simulink subsystem "Wind_Table"  (R2023b)
settings: Solver=VariableStepAuto  StartTime=0.0  StopTime=10.0  RelTol=1e-3
undefined symbols (not defined in the file): time0, wind_direction_table, wind_speed_table
libraries: sharedtransform x1
settings Model: Creator=thatf  LastModifiedBy=thatf

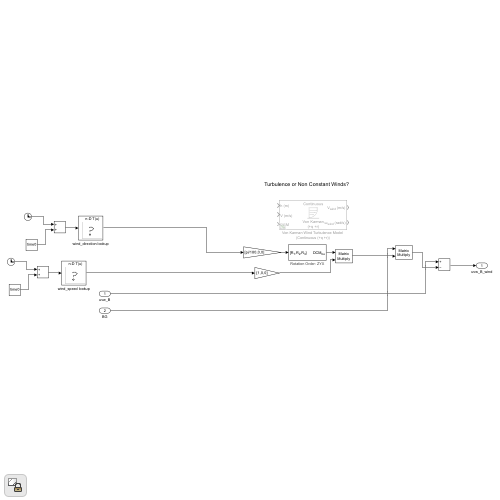
[thumbnail: Simulink's stored preview of the top-level diagram]
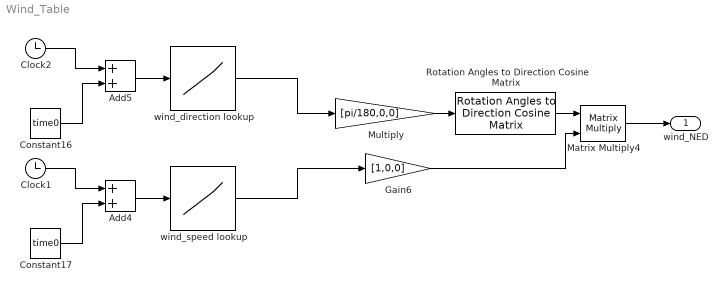
== system Wind_Table ==
  Add4 : Sum
  Add5 : Sum
  Clock1 : Clock
  Clock2 : Clock
  Constant16 : Constant  Value=time0
  Constant17 : Constant  Value=time0
  Gain6 : Gain  Gain=[1,0,0]
  Matrix Multiply4 : Product  Multiplication=Matrix(*)
  Multiply : Gain  Gain=[pi/180,0,0]
  Rotation Angles to Direction Cosine Matrix : sharedtransform/Rotation Angles to Direction Cosine Matrix  rotationOrder=ZYX  aMode=aMode
  wind_direction lookup : Lookup_n-D  NumberOfTableDimensions=1  BreakpointsForDimension1=wind_direction_table(:,1)  Table=wind_direction_table(:,2)  InternalRulePriority=Speed  RndMeth=Simplest
  wind_speed lookup : Lookup_n-D  NumberOfTableDimensions=1  BreakpointsForDimension1=wind_speed_table(:,1)  Table=wind_speed_table(:,2)  InternalRulePriority=Speed  RndMeth=Simplest
  wind_NED : Outport
  wires:
  Rotation Angles to Direction Cosine Matrix/1 -> Matrix Multiply4/1
  Gain6/1 -> Matrix Multiply4/2
  Multiply/1 -> Rotation Angles to Direction Cosine Matrix/1
  Constant17/1 -> Add4/2
  wind_speed lookup/1 -> Gain6/1
  wind_direction lookup/1 -> Multiply/1
  Add5/1 -> wind_direction lookup/1
  Add4/1 -> wind_speed lookup/1
  Constant16/1 -> Add5/2
  Clock2/1 -> Add5/1
  Clock1/1 -> Add4/1
  Matrix Multiply4/1 -> wind_NED/1
